simulink model "sampleModel1725"  (R2023a)
settings: Solver=VariableStepAuto  StartTime=0.0  StopTime=10.0  RelTol=1e-3
libraries: hdlsllib x4, simulink x3
settings Model: Creator=user1  LastModifiedBy=user1

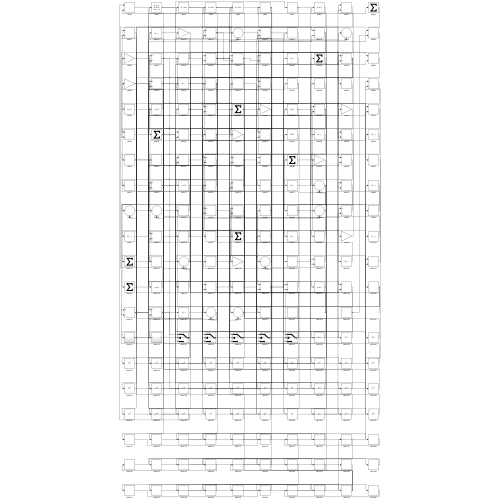
[thumbnail: Simulink's stored preview of the top-level diagram]
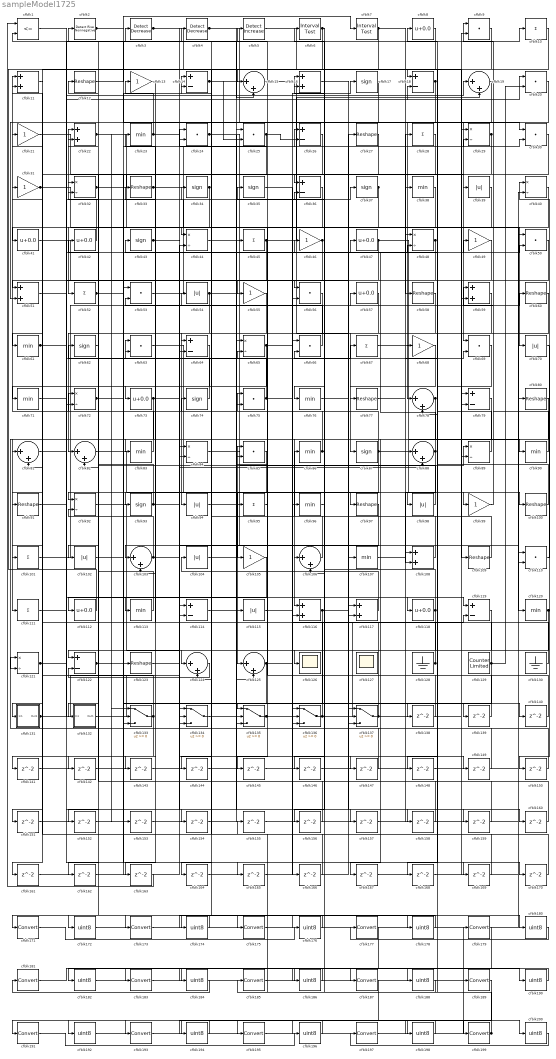
== system sampleModel1725 ==
  cfblk1 : RelationalOperator  Operator=<=  OutDataTypeStr=boolean  InputSameDT=off
  cfblk{10,28,45,52,67,95,101,111} (8 alike) : Sum  Inputs=+
  cfblk{12,27,33,58,60,77,80,91,97,100,109,123} (12 alike) : Reshape
  cfblk{39,54,70,94,98,102,104,115} (8 alike) : Abs  SaturateOnIntegerOverflow=off
  cfblk{15,19,78,81..82,88,103,106,124..125} (10 alike) : Sum  Inputs=|++
  cfblk{13,21,31,46,49,55,68,99,105} (9 alike) : Gain
  cfblk{23,38,61,71,76,83,86,90,96,107,113,120} (12 alike) : MinMax
  cfblk{11,16,22,51,59,108,116..117} (8 alike) : Sum
  cfblk{9,20,24..25,30,50,53,56,63,66,69,75,85,110} (14 alike) : DotProduct  OutDataTypeStr=Inherit: Inherit via internal rule
  cfblk{8,41..42,47,57,73,112,118} (8 alike) : Bias  Bias=0.0  SaturateOnIntegerOverflow=off
  cfblk{14,18,26,36,64,79,114,119,122} (9 alike) : Sum  Inputs=+-
  cfblk{29,32,40,44,48,65,72,84,89,92,121} (11 alike) : Product  Inputs=*/  RndMeth=Zero  SaturateOnIntegerOverflow=on
  cfblk126 : Scope
  cfblk127 : Scope
      settings: Floating=on
  cfblk128 : Ground
  cfblk129 : hdlsllib/Sources/Counter Limited  uplimit=7  tsamp=-1
  cfblk130 : Ground
  cfblk131 : Subsystem
      settings: LibrarySourceBlock=|
      | hdlsllib/Ports &
      | Subsystems/Subsystem
  cfblk132 : Subsystem
      settings: LibrarySourceBlock=|
      | hdlsllib/Ports &
      | Subsystems/Subsystem
  cfblk{133..137} (5 alike) : Switch  SaturateOnIntegerOverflow=off  InputSameDT=off
  cfblk{138..170} (33 alike) : Delay  SampleTime=1
  cfblk{17,34..35,37,43,62,74,87,93} (9 alike) : Signum
  cfblk{171,173,175,177,179,181,183,185,187,189,191,193,195,197,199} (15 alike) : DataTypeConversion  SaturateOnIntegerOverflow=off  RndMeth=Floor
  cfblk{172,174,176,178,180,182,184,186,188,190,192,194,196,198,200} (15 alike) : DataTypeConversion  OutDataTypeStr=uint8  SaturateOnIntegerOverflow=off  RndMeth=Floor
  cfblk2 : hdlsllib/Logic and Bit Operations/Detect Rise Nonnegative  vinit=0  OutDataTypeStr=boolean
  cfblk3 : simulink/Logic and Bit Operations/Detect Decrease  vinit=0.0  OutDataTypeStr=boolean
      settings: LibrarySourceBlock=|
      | hdlsllib/Logic and Bit
      | Operations/Detect
      | Decrease
  cfblk4 : simulink/Logic and Bit Operations/Detect Decrease  vinit=0.0  OutDataTypeStr=boolean
      settings: LibrarySourceBlock=|
      | hdlsllib/Logic and Bit
      | Operations/Detect
      | Decrease
  cfblk5 : simulink/Logic and Bit Operations/Detect Increase  vinit=0.0  OutDataTypeStr=boolean
      settings: LibrarySourceBlock=|
      | hdlsllib/Logic and Bit
      | Operations/Detect
      | Increase
  cfblk6 : hdlsllib/Logic and Bit Operations/Interval Test  IntervalClosedRight=on  uplimit=0.5  IntervalClosedLeft=on  lowlimit=-0.5  OutDataTypeStr=boolean
  cfblk7 : hdlsllib/Logic and Bit Operations/Interval Test  IntervalClosedRight=on  uplimit=0.5  IntervalClosedLeft=on  lowlimit=-0.5  OutDataTypeStr=boolean
  wires:
  cfblk120/1 -> cfblk122/1, cfblk135/2
  cfblk83/1 -> cfblk11/1
  cfblk67/1 -> cfblk90/1
  cfblk24/1 -> cfblk89/1, cfblk136/2, cfblk18/2
  cfblk61/1 -> cfblk20/1, cfblk165/1
  cfblk14/1 -> cfblk69/1, cfblk25/2
  cfblk100/1 -> cfblk43/1
  cfblk53/1 -> cfblk37/1
  cfblk47/1 -> cfblk99/1, cfblk113/1
  cfblk40/1 -> cfblk52/1
  cfblk93/1 -> cfblk42/1, cfblk149/1
  cfblk112/1 -> cfblk18/1
  cfblk37/1 -> cfblk126/1, cfblk132/1(In1)
  cfblk125/1 -> cfblk17/1, cfblk133/2
  cfblk18/1 -> cfblk78/1, cfblk51/2
  cfblk104/1 -> cfblk85/1
  cfblk101/1 -> cfblk27/1
  cfblk41/1 -> cfblk123/1
  cfblk49/1 -> cfblk55/1
  cfblk96/1 -> cfblk16/1
  cfblk89/1 -> cfblk66/2
  cfblk42/1 -> cfblk22/1
  cfblk85/1 -> cfblk92/1
  cfblk25/1 -> cfblk73/1, cfblk26/2
  cfblk82/1 -> cfblk100/1
  cfblk65/1 -> cfblk102/1, cfblk140/1
  cfblk7/1 -> cfblk58/1, cfblk164/1
  cfblk9/1 -> cfblk68/1
  cfblk56/1 -> cfblk82/1
  cfblk44/1 -> cfblk117/2
  cfblk79/1 -> cfblk111/1
  cfblk107/1 -> cfblk28/1
  cfblk6/1 -> cfblk51/1, cfblk76/1
  cfblk137/1 -> cfblk54/1, cfblk29/1, cfblk81/2
  cfblk22/1 -> cfblk70/1, cfblk133/1
  cfblk74/1 -> cfblk32/1
  cfblk58/1 -> cfblk87/1
  cfblk136/1 -> cfblk79/1, cfblk4/1
  cfblk130/1 -> cfblk63/1
  cfblk55/1 -> cfblk112/1
  cfblk75/1 -> cfblk63/2, cfblk32/2, cfblk29/2
  cfblk103/1 -> cfblk72/1, cfblk57/1, cfblk60/1
  cfblk110/1 -> cfblk40/1
  cfblk52/1 -> cfblk14/1, cfblk170/1
  cfblk29/1 -> cfblk124/1, cfblk36/1, cfblk133/3
  cfblk113/1 -> cfblk62/1
  cfblk21/1 -> cfblk137/1
  cfblk17/1 -> cfblk24/2
  cfblk4/1 -> cfblk109/1, cfblk15/2
  cfblk114/1 -> cfblk45/1
  cfblk20/1 -> cfblk83/1
  cfblk123/1 -> cfblk135/1
  cfblk92/1 -> cfblk134/1
  cfblk98/1 -> cfblk2/1
  cfblk15/1 -> cfblk107/1
  cfblk60/1 -> cfblk94/1
  cfblk68/1 -> cfblk77/1
  cfblk81/1 -> cfblk67/1
  cfblk78/1 -> cfblk116/1, cfblk167/1
  cfblk63/1 -> cfblk125/1
  cfblk23/1 -> cfblk13/1, cfblk88/2
  cfblk19/1 -> cfblk91/1
  cfblk111/1 -> cfblk49/1
  cfblk88/1 -> cfblk47/1, cfblk108/2
  cfblk84/1 -> cfblk110/2
  cfblk121/1 -> cfblk19/1, cfblk50/2, cfblk169/1
  cfblk99/1 -> cfblk9/1
  cfblk45/1 -> cfblk19/2, cfblk64/2
  cfblk46/1 -> cfblk136/3, cfblk142/1
  cfblk31/1 -> cfblk101/1, cfblk120/1, cfblk160/1
  cfblk108/1 -> cfblk86/1
  cfblk51/1 -> cfblk3/1
  cfblk106/1 -> cfblk75/1
  cfblk62/1 -> cfblk12/1
  cfblk91/1 -> cfblk65/2
  cfblk73/1 -> cfblk114/2, cfblk121/2
  cfblk97/1 -> cfblk103/1
  cfblk48/1 -> cfblk115/1, cfblk61/1
  cfblk8/1 -> cfblk72/2
  cfblk54/1 -> cfblk10/1, cfblk93/1
  cfblk71/1 -> cfblk118/1
  cfblk72/1 -> cfblk119/1, cfblk154/1
  cfblk122/1 -> cfblk26/1, cfblk152/1, cfblk153/1
  cfblk115/1 -> cfblk96/1
  cfblk11/1 -> cfblk71/1
  cfblk128/1 -> cfblk16/2, cfblk33/1
  cfblk33/1 -> cfblk9/2, cfblk79/2
  cfblk77/1 -> cfblk38/1
  cfblk135/1 -> cfblk119/2, cfblk147/1
  cfblk66/1 -> cfblk53/2
  cfblk117/1 -> cfblk104/1
  cfblk36/1 -> cfblk105/1
  cfblk2/1 -> cfblk30/1, cfblk7/1
  cfblk34/1 -> cfblk44/1, cfblk81/1
  cfblk118/1 -> cfblk35/1, cfblk124/2
  cfblk131/1(Out1) -> cfblk44/2, cfblk34/1
  cfblk32/1 -> cfblk39/1, cfblk36/2
  cfblk87/1 -> cfblk23/1, cfblk69/2, cfblk163/1
  cfblk132/1(Out1) -> cfblk84/2
  cfblk90/1 -> cfblk59/1
  cfblk43/1 -> cfblk106/1, cfblk97/1
  cfblk50/1 -> cfblk131/1(In1)
  cfblk133/1 -> cfblk31/1, cfblk161/1
  cfblk3/1 -> cfblk15/1, cfblk158/1
  cfblk16/1 -> cfblk98/1
  cfblk1/1 -> cfblk56/1
  cfblk59/1 -> cfblk95/1
  cfblk124/1 -> cfblk122/2
  cfblk30/1 -> cfblk64/1
  cfblk28/1 -> cfblk103/2
  cfblk5/1 -> cfblk59/2
  cfblk86/1 -> cfblk21/1, cfblk146/1
  cfblk12/1 -> cfblk5/1
  cfblk129/1 -> cfblk85/2, cfblk134/3, cfblk20/2
  cfblk109/1 -> cfblk74/1
  cfblk116/1 -> cfblk48/2, cfblk30/2, cfblk135/3
  cfblk10/1 -> cfblk41/1
  cfblk134/1 -> cfblk46/1
  cfblk69/1 -> cfblk138/1
  cfblk138/1 -> cfblk24/1
  cfblk102/1 -> cfblk139/1
  cfblk139/1 -> cfblk65/1
  cfblk140/1 -> cfblk1/2
  cfblk64/1 -> cfblk141/1
  cfblk141/1 -> cfblk114/1
  cfblk142/1 -> cfblk125/2
  cfblk13/1 -> cfblk143/1
  cfblk143/1 -> cfblk84/1
  cfblk38/1 -> cfblk144/1
  cfblk144/1 -> cfblk88/1
  cfblk95/1 -> cfblk145/1
  cfblk145/1 -> cfblk40/2
  cfblk146/1 -> cfblk108/1
  cfblk147/1 -> cfblk82/2
  cfblk119/1 -> cfblk148/1
  cfblk148/1 -> cfblk78/2
  cfblk149/1 -> cfblk66/1
  cfblk70/1 -> cfblk150/1
  cfblk150/1 -> cfblk121/1
  cfblk27/1 -> cfblk151/1
  cfblk151/1 -> cfblk48/1
  cfblk152/1 -> cfblk75/2
  cfblk153/1 -> cfblk136/1
  cfblk154/1 -> cfblk137/3
  cfblk155/1 -> cfblk56/2
  cfblk57/1 -> cfblk156/1
  cfblk156/1 -> cfblk22/2
  cfblk94/1 -> cfblk157/1
  cfblk157/1 -> cfblk110/1
  cfblk158/1 -> cfblk137/2
  cfblk76/1 -> cfblk159/1
  cfblk159/1 -> cfblk25/1
  cfblk160/1 -> cfblk92/2
  cfblk161/1 -> cfblk134/2
  cfblk105/1 -> cfblk162/1
  cfblk162/1 -> cfblk53/1
  cfblk163/1 -> cfblk1/1
  cfblk164/1 -> cfblk116/2
  cfblk165/1 -> cfblk117/1
  cfblk35/1 -> cfblk166/1
  cfblk166/1 -> cfblk11/2
  cfblk167/1 -> cfblk89/2
  cfblk39/1 -> cfblk168/1
  cfblk168/1 -> cfblk50/1
  cfblk169/1 -> cfblk14/2
  cfblk170/1 -> cfblk106/2
  cfblk26/1 -> cfblk172/1
  cfblk172/1 -> cfblk80/1
  cfblk80/1 -> cfblk174/1
  cfblk174/1 -> cfblk171/1
  cfblk171/1 -> cfblk176/1
  cfblk176/1 -> cfblk173/1
  cfblk173/1 -> cfblk178/1
  cfblk178/1 -> cfblk175/1
  cfblk175/1 -> cfblk180/1
  cfblk180/1 -> cfblk177/1
  cfblk177/1 -> cfblk182/1
  cfblk182/1 -> cfblk179/1
  cfblk179/1 -> cfblk184/1
  cfblk184/1 -> cfblk181/1
  cfblk181/1 -> cfblk186/1
  cfblk186/1 -> cfblk183/1
  cfblk183/1 -> cfblk188/1
  cfblk188/1 -> cfblk185/1
  cfblk185/1 -> cfblk190/1
  cfblk190/1 -> cfblk187/1
  cfblk187/1 -> cfblk192/1
  cfblk192/1 -> cfblk189/1
  cfblk189/1 -> cfblk194/1
  cfblk194/1 -> cfblk191/1
  cfblk191/1 -> cfblk196/1
  cfblk196/1 -> cfblk193/1
  cfblk197/1 -> cfblk199/1
  cfblk193/1 -> cfblk198/1
  cfblk198/1 -> cfblk195/1
  cfblk199/1 -> cfblk155/1, cfblk6/1, cfblk8/1
  cfblk195/1 -> cfblk200/1
  cfblk200/1 -> cfblk197/1

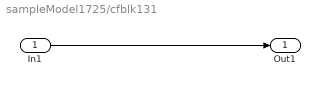
== system sampleModel1725/cfblk131 ==
  In1 : Inport
  Out1 : Outport
  wires:
  In1/1 -> Out1/1

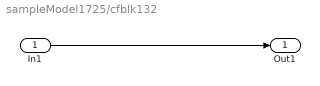
== system sampleModel1725/cfblk132 ==
  In1 : Inport
  Out1 : Outport
  wires:
  In1/1 -> Out1/1
